simulink model "Double_Tank_sim"  (Simulink 10.2)
settings: Solver=VariableStepAuto  StartTime=0.0  StopTime=100  RelTol=1e-3
values from neighbouring files (symbols this model uses):
  K = acker(A,B,poles)    [double_tank_init.m]
  V = -1/(C*inv(A-B*K)*B)    [double_tank_init.m]
  x_init = [0.1 0.15]    [double_tank_init.m]
libraries: mci_models x2
settings Model: Creator=12064  LastModifiedBy=12064  MultiThreadCoSim=auto
settings DataIOCC: SaveFormat=Dataset  SignalLoggingSaveFormat=Dataset  ReturnWorkspaceOutputs=on
settings OptimizationCC: LifeSpan=auto
settings DebuggingCC: UnderspecifiedInitializationDetection=Simplified  MergeDetectMultiDrivingBlocksExec=error  FcnCallInpInsideContextMsg=error  UnconnectedInputMsg=none  UnconnectedOutputMsg=none  UnconnectedLineMsg=none  SFUnexpectedBacktrackingDiag=error  SFNoUnconditionalDefaultTransitionDiag=error  SFExecutionAtInitializationDiag=warning  ArithmeticOperatorsInVariantConditions=error
settings HardwareCC: ProdBitPerPointer=64  ProdBitPerSizeT=64  ProdBitPerPtrDiffT=64  ProdLargestAtomicFloat=Float  ProdIntDivRoundTo=Zero  ProdEndianess=LittleEndian  ProdWordSize=64  ProdHWDeviceType=Intel->x86-64 (Windows64)
settings ModelReferenceCC: EnableRefExpFcnMdlSchedulingChecks=off  PropagateSignalLabelsOutOfModel=on
settings SFSimCC: SimUseLocalCustomCode=on  CustomCodeUndefinedFunction=FilterOut
settings RTWCC: RTWUseLocalCustomCode=on
settings CodeAppCC: StateflowObjectComments=off
settings GRTTargetCC: TargetLangStandard=C99 (ISO)  CombineOutputUpdateFcns=on  GRTInterface=off
settings ConfigComp: CovMetricSettings=dwe  CovSaveCumulativeToWorkspaceVar=off  CovSaveSingleToWorkspaceVar=off  CovExternalEMLEnable=on

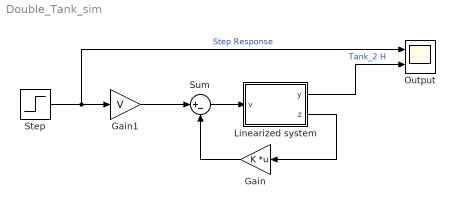
== system Double_Tank_sim ==
  Gain : Gain  Gain=K  Multiplication=Matrix(K*u)
  Gain1 : Gain  Gain=V
  Linearized system : Subsystem
  Output : Scope  NumInputPorts=2
  Step : Step  Time=10  Before=.05  After=.1  SampleTime=0
  Sum : Sum  Inputs=|+-
  wires:
  Linearized system/1(y) -> Output/2  "Tank_2 H"
  Sum/1 -> Linearized system/1(v)
  Linearized system/2(z) -> Gain/1
  Gain/1 -> Sum/2
  Gain1/1 -> Sum/1
  Step/1 -> Output/1, Gain1/1  "Step Response"

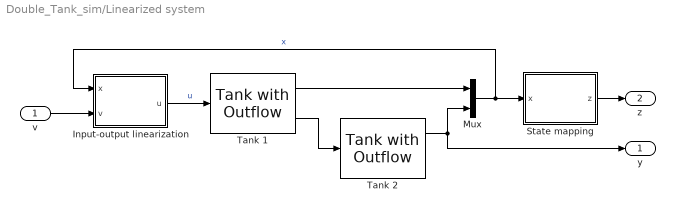
== system Double_Tank_sim/Linearized system ==
  v : Inport
  Input-output linearization : MATLAB Function  TreatAsAtomicUnit=on
  Mux : Mux  Inputs=2
  State mapping : MATLAB Function  TreatAsAtomicUnit=on
  Tank 1 : mci_models/Fluid Systems/Tank with Outflow  At=p.At  Ao=p.Ao  rho=p.rho  zeta=p.zeta  g=9.81  h0=x_init(1)
  Tank 2 : mci_models/Fluid Systems/Tank with Outflow  At=p.At  Ao=p.Ao  rho=p.rho  zeta=p.zeta  g=9.81  h0=x_init(2)
  y : Outport
  z : Outport  Port=2
  wires:
  Tank 1/2 -> Tank 2/1
  Input-output linearization/1(u) -> Tank 1/1  "u"
  v/1 -> Input-output linearization/2(v)
  State mapping/1(z) -> z/1
  Mux/1 -> State mapping/1(x), Input-output linearization/1(x)  "x"
  Tank 1/1 -> Mux/1
  Tank 2/1 -> y/1, Mux/2

== matlab function Linearized system/State mapping ==
  data: x input double; z output double; p parameter double
function z = fcn(x,p)
%#codegen
z = 0*x; % assignment before subscripting
z(1) = x(2);
z(2) = p.a*sqrt(x(1))-p.a*sqrt(x(2));

== matlab function Linearized system/Input-output linearization ==
  data: x input double; v input double; u output double; p parameter double
function u = fcn(x,v,p)
u = 0;
u = p.rho*p.At*sqrt(x(1))*(2*v/p.a+...
    p.a*sqrt(x(1))/sqrt(x(2)));
